simulink model "prochazkaModelWithVM"  (R2022b)
settings: Solver=VariableStepAuto  StartTime=0.0  StopTime=10.0  MaxStep=0.2  RelTol=1e-3
settings Model: SimulationMode=accelerator  Creator=migpa  LastModifiedBy=migpa
settings SolverCC: AlgebraicLoopSolver=TrustRegion
settings DebuggingCC: UnconnectedInputMsg=warning  UnconnectedOutputMsg=warning  UnconnectedLineMsg=warning  SFMachineParentedDataDiag=warning
settings ModelReferenceCC: EnableRefExpFcnMdlSchedulingChecks=on
settings RTWCC: DLArmComputeVersion=19.05

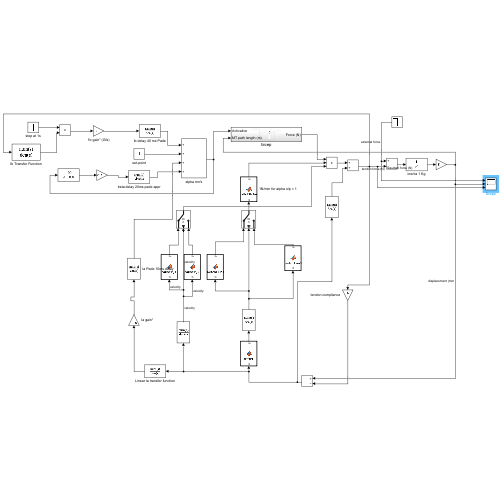
[thumbnail: Simulink's stored preview of the top-level diagram]
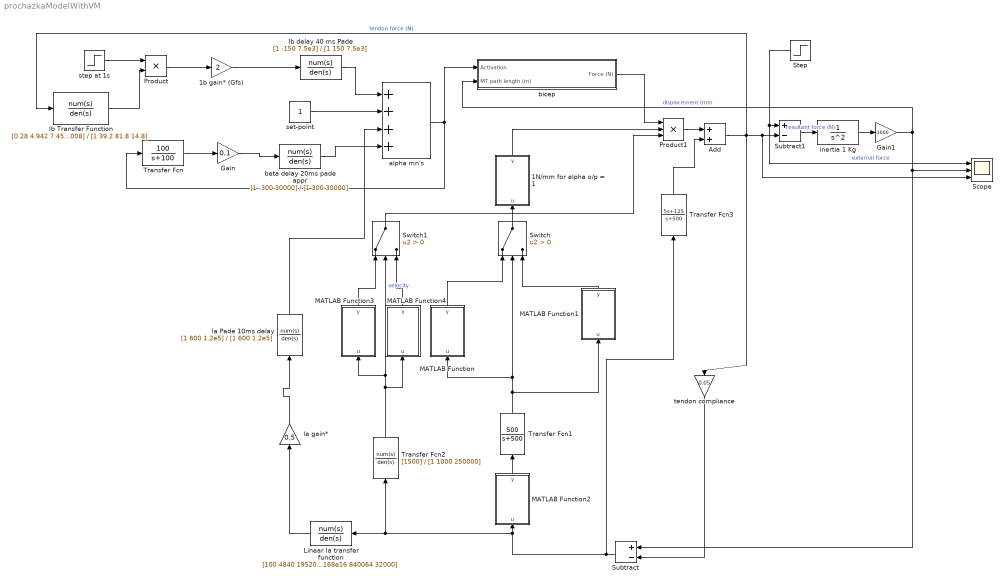
== system prochazkaModelWithVM ==
  1N/mm for alpha o/p = 1 : MATLAB Function  TreatAsAtomicUnit=on
  1b gain* (Gfs) : Gain  Gain=2
  Add : Sum
  Gain : Gain  Gain=0.1
  Gain1 : Gain  Gain=1000
  Ia Pade 10ms delay : TransferFcn  Numerator=[1 600 1.2e5]  Denominator=[1 600 1.2e5]
  Ia gain* : Gain  Gain=0.5
  Ib Transfer Function : TransferFcn  Numerator=[0.28 4.942 7.455 1.008]  Denominator=[1 39.2 81.8 14.8]
  Ib delay 40 ms Pade : TransferFcn  Numerator=[1 -150 7.5e3]  Denominator=[1 150 7.5e3]
  Linear Ia transfer function : TransferFcn  Numerator=[100 4840 19520 7040]  Denominator=[1 2000.84 1.00168e16 840064 32000]
  MATLAB Function : MATLAB Function  TreatAsAtomicUnit=on
  MATLAB Function1 : MATLAB Function  TreatAsAtomicUnit=on
  MATLAB Function2 : MATLAB Function  TreatAsAtomicUnit=on
  MATLAB Function3 : MATLAB Function  TreatAsAtomicUnit=on
  MATLAB Function4 : MATLAB Function  TreatAsAtomicUnit=on
  Product : Product
  Product1 : Product  Inputs=3
  Scope : Scope  NumInputPorts=3
  Step : Step  Before=30  After=0  SampleTime=0
  Subtract : Sum  Inputs=+-
  Subtract1 : Sum  Inputs=+-
  Switch : Switch  Criteria=u2 > Threshold  SaturateOnIntegerOverflow=off  InputSameDT=off
  Switch1 : Switch  Criteria=u2 > Threshold  SaturateOnIntegerOverflow=off  InputSameDT=off
  Transfer Fcn : TransferFcn  Numerator=[100]  Denominator=[1 100]
  Transfer Fcn1 : TransferFcn  Numerator=[500]  Denominator=[1 500]
  Transfer Fcn2 : TransferFcn  Numerator=[1500]  Denominator=[1 1000 250000]
  Transfer Fcn3 : TransferFcn  Numerator=[5 125]  Denominator=[1 500]
  alpha mn's : Sum  Inputs=++++
  beta delay 20ms pade appr : TransferFcn  Numerator=[1 -300 30000]  Denominator=[1 300 30000]
  bicep : Subsystem
  inertia 1 Kg : TransferFcn  Denominator=[1 0 0]
  set-point : Constant
  step at 1s : Step  SampleTime=0
  tendon compliance : Gain  Gain=0.05
  wires:
  Transfer Fcn/1 -> Gain/1
  step at 1s/1 -> Product/1
  Ib Transfer Function/1 -> Product/2
  set-point/1 -> alpha mn's/2
  Product/1 -> 1b gain* (Gfs)/1
  1b gain* (Gfs)/1 -> Ib delay 40 ms Pade/1
  Gain/1 -> beta delay 20ms pade appr/1
  alpha mn's/1 -> bicep/1(Activation), Transfer Fcn/1
  Switch/1 -> 1N/mm for alpha o/p = 1/1(u)
  bicep/1(Force (N)) -> Product1/1
  MATLAB Function/1(y) -> Switch/1
  MATLAB Function1/1(y) -> Switch/3
  Transfer Fcn1/1 -> MATLAB Function1/1(u), MATLAB Function/1(u), Switch/2
  MATLAB Function2/1(y) -> Transfer Fcn1/1
  Subtract/1 -> Transfer Fcn2/1, Linear Ia transfer function/1, MATLAB Function2/1(u), Transfer Fcn3/1
  tendon compliance/1 -> Subtract/2
  Ia gain*/1 -> Ia Pade 10ms delay/1
  Linear Ia transfer function/1 -> Ia gain*/1
  Ia Pade 10ms delay/1 -> alpha mn's/3
  1N/mm for alpha o/p = 1/1(y) -> Product1/2
  Transfer Fcn2/1 -> MATLAB Function4/1(u), MATLAB Function3/1(u), Switch1/2  "velocity"
  MATLAB Function3/1(y) -> Switch1/1
  MATLAB Function4/1(y) -> Switch1/3
  Switch1/1 -> Product1/3
  Product1/1 -> Add/1
  Transfer Fcn3/1 -> Add/2
  Add/1 -> tendon compliance/1, Ib Transfer Function/1, Scope/3, Subtract1/2  "tendon force (N)"
  Subtract1/1 -> inertia 1 Kg/1  "resultant force (N)"
  inertia 1 Kg/1 -> Gain1/1
  Gain1/1 -> Subtract/1, Scope/2, bicep/2(MT path length (m))  "displacement (mm"
  Step/1 -> Scope/1, Subtract1/1  "external force"
  Ib delay 40 ms Pade/1 -> alpha mn's/1
  beta delay 20ms pade appr/1 -> alpha mn's/4

== system prochazkaModelWithVM/bicep ==
  Activation : Inport
  MT path length (m) : Inport  Port=2
  Convert m to cm : Gain  Gain=100
  Recruitment : Subsystem
  fascicles (CE & PE) : Subsystem
  muscle mass : Subsystem
  series elastic element : Subsystem
  Force (N) : Outport
  wires:
  MT path length (m)/1 -> Convert m to cm/1
  series elastic element/1(Fse (N)) -> muscle mass/2(Fse (N)), Force (N)/1
  fascicles (CE & PE)/1(Force (N)) -> muscle mass/1(Fce (N))
  muscle mass/2(Lce (L0)) -> fascicles (CE & PE)/2(Length (L0)), series elastic element/2(Lce (L0))
  muscle mass/1(Vce (L0/s)) -> fascicles (CE & PE)/3(Velocity (L0/s))
  Recruitment/1(Frequencies (f0.5)) -> fascicles (CE & PE)/1(Frequencies (f0.5))
  Convert m to cm/1 -> series elastic element/1(Path (cm)), muscle mass/3(Path length [for init] (cm))
  Activation/1 -> Recruitment/1(Activation)

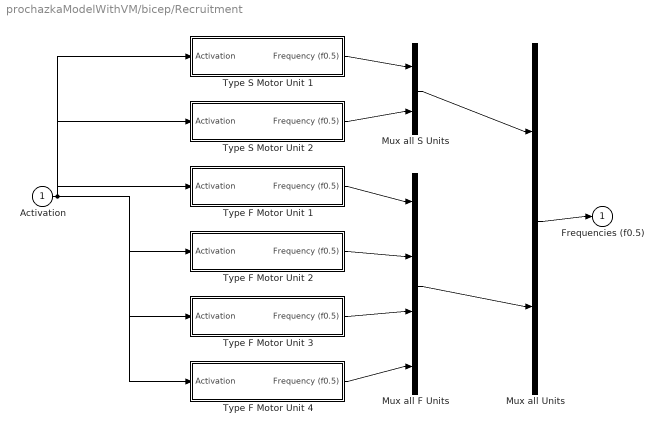
== system prochazkaModelWithVM/bicep/Recruitment ==
  Activation : Inport
  Mux all F Units : Mux
  Mux all S Units : Mux  Inputs=2
  Mux all Units : Mux  Inputs=2
  Type F Motor Unit 1 : Subsystem
  Type F Motor Unit 2 : Subsystem
  Type F Motor Unit 3 : Subsystem
  Type F Motor Unit 4 : Subsystem
  Type S Motor Unit 1 : Subsystem
  Type S Motor Unit 2 : Subsystem
  Frequencies (f0.5) : Outport
  wires:
  Activation/1 -> Type S Motor Unit 1/1(Activation), Type S Motor Unit 2/1(Activation), Type F Motor Unit 1/1(Activation), Type F Motor Unit 2/1(Activation), Type F Motor Unit 3/1(Activation), Type F Motor Unit 4/1(Activation)
  Type S Motor Unit 1/1(Frequency (f0.5)) -> Mux all S Units/1
  Type S Motor Unit 2/1(Frequency (f0.5)) -> Mux all S Units/2
  Mux all S Units/1 -> Mux all Units/1
  Type F Motor Unit 1/1(Frequency (f0.5)) -> Mux all F Units/1
  Type F Motor Unit 2/1(Frequency (f0.5)) -> Mux all F Units/2
  Type F Motor Unit 3/1(Frequency (f0.5)) -> Mux all F Units/3
  Type F Motor Unit 4/1(Frequency (f0.5)) -> Mux all F Units/4
  Mux all F Units/1 -> Mux all Units/2
  Mux all Units/1 -> Frequencies (f0.5)/1

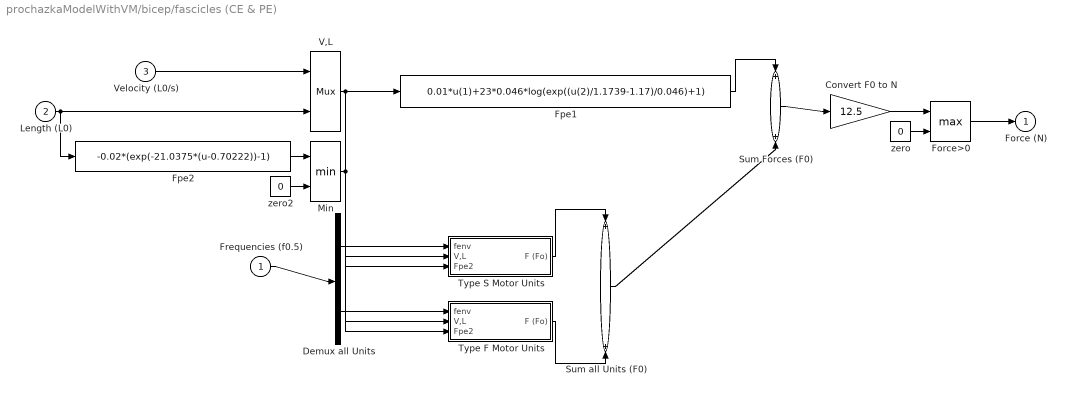
== system prochazkaModelWithVM/bicep/fascicles (CE & PE) ==
  Frequencies (f0.5) : Inport
  Length (L0) : Inport  Port=2
  Velocity (L0/s) : Inport  Port=3
  Convert F0 to N : Gain  Gain=12.5
  Demux all Units : Demux  Outputs="[2  4]"
  Force>0 : MinMax  Function=max  Inputs=2
  Fpe1 : Fcn  Expr=0.01*u(1)+23*0.046*log(exp((u(2)/1.1739-1.17)/0.046)+1)
  Fpe2 : Fcn  Expr=-0.02*(exp(-21.0375*(u-0.70222))-1)
  Min : MinMax  Inputs=2
  Sum Forces (F0) : Sum  Inputs=2
  Sum all Units (F0) : Sum
  Type F Motor Units : Subsystem
  Type S Motor Units : Subsystem
  V,L : Mux  Inputs=2
  zero : Constant  Value=0
  zero2 : Constant  Value=0
  Force (N) : Outport
  wires:
  Demux all Units/1 -> Type S Motor Units/1(fenv)
  V,L/1 -> Type S Motor Units/2(V,L), Type F Motor Units/2(V,L), Fpe1/1
  Min/1 -> Type S Motor Units/3(Fpe2), Type F Motor Units/3(Fpe2)
  Type S Motor Units/1(F (Fo)) -> Sum all Units (F0)/1
  Demux all Units/2 -> Type F Motor Units/1(fenv)
  Type F Motor Units/1(F (Fo)) -> Sum all Units (F0)/2
  Length (L0)/1 -> Fpe2/1, V,L/2
  Velocity (L0/s)/1 -> V,L/1
  Fpe2/1 -> Min/1
  zero2/1 -> Min/2
  Frequencies (f0.5)/1 -> Demux all Units/1
  Convert F0 to N/1 -> Force>0/1
  zero/1 -> Force>0/2
  Force>0/1 -> Force (N)/1
  Fpe1/1 -> Sum Forces (F0)/1
  Sum all Units (F0)/1 -> Sum Forces (F0)/2
  Sum Forces (F0)/1 -> Convert F0 to N/1

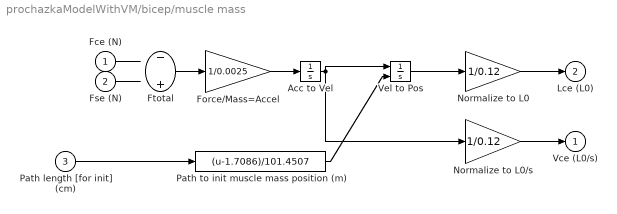
== system prochazkaModelWithVM/bicep/muscle mass ==
  Fce (N) : Inport
  Fse (N) : Inport  Port=2
  Path length [for init] (cm) : Inport  Port=3
  Acc to Vel : Integrator
  Force/Mass=Accel : Gain  Gain=1/0.0025
  Ftotal : Sum  Inputs=-+
  Normalize to L0 : Gain  Gain=1/0.12
  Normalize to L0/s : Gain  Gain=1/0.12
  Path to init muscle mass position (m) : Fcn  Expr=(u-1.7086)/101.4507
  Vel to Pos : Integrator  InitialConditionSource=external
  Vce (L0/s) : Outport
  Lce (L0) : Outport  Port=2
  wires:
  Ftotal/1 -> Force/Mass=Accel/1
  Force/Mass=Accel/1 -> Acc to Vel/1
  Acc to Vel/1 -> Vel to Pos/1, Normalize to L0/s/1
  Path length [for init] (cm)/1 -> Path to init muscle mass position (m)/1
  Path to init muscle mass position (m)/1 -> Vel to Pos/2
  Vel to Pos/1 -> Normalize to L0/1
  Fce (N)/1 -> ?
  Normalize to L0/1 -> Lce (L0)/1
  Fse (N)/1 -> ?
  Normalize to L0/s/1 -> Vce (L0/s)/1

== system prochazkaModelWithVM/bicep/series elastic element ==
  Path (cm) : Inport
  Lce (L0) : Inport  Port=2
  Convert Lce to Lse : Sum  Inputs=+-
  Convert to N : Gain  Gain=12.5
  Convert to cm : Gain  Gain=12
  Fse : Fcn  Expr=27.8*0.0047*log(exp((u(1)-0.964)/0.0047)+1)
  Normalize to L0T : Gain  Gain=1/2
  Fse (N) : Outport
  wires:
  Fse/1 -> Convert to N/1
  Normalize to L0T/1 -> Fse/1
  Convert Lce to Lse/1 -> Normalize to L0T/1
  Convert to N/1 -> Fse (N)/1
  Lce (L0)/1 -> Convert to cm/1
  Convert to cm/1 -> ?
  Path (cm)/1 -> ?

== system prochazkaModelWithVM/bicep/Recruitment/Type F Motor Unit 1 ==
  Activation : Inport
  Reached recruitment threshold? : Switch  Threshold=0.5
  determine frequency : Fcn  Expr=((2-0.5)/(1-(0.5)))*(u(1)-(0.5))+0.5
  zero : Constant  Value=0
  Frequency (f0.5) : Outport
  wires:
  Activation/1 -> Reached recruitment threshold?/2, determine frequency/1
  Reached recruitment threshold?/1 -> Frequency (f0.5)/1
  determine frequency/1 -> Reached recruitment threshold?/1
  zero/1 -> Reached recruitment threshold?/3

== system prochazkaModelWithVM/bicep/Recruitment/Type F Motor Unit 2 ==
  Activation : Inport
  Reached recruitment threshold? : Switch  Threshold=0.6
  determine frequency : Fcn  Expr=((2-0.5)/(1-(0.6)))*(u(1)-(0.6))+0.5
  zero : Constant  Value=0
  Frequency (f0.5) : Outport
  wires:
  Activation/1 -> Reached recruitment threshold?/2, determine frequency/1
  Reached recruitment threshold?/1 -> Frequency (f0.5)/1
  determine frequency/1 -> Reached recruitment threshold?/1
  zero/1 -> Reached recruitment threshold?/3

== system prochazkaModelWithVM/bicep/Recruitment/Type F Motor Unit 3 ==
  Activation : Inport
  Reached recruitment threshold? : Switch  Threshold=0.7
  determine frequency : Fcn  Expr=((2-0.5)/(1-(0.7)))*(u(1)-(0.7))+0.5
  zero : Constant  Value=0
  Frequency (f0.5) : Outport
  wires:
  Activation/1 -> Reached recruitment threshold?/2, determine frequency/1
  Reached recruitment threshold?/1 -> Frequency (f0.5)/1
  determine frequency/1 -> Reached recruitment threshold?/1
  zero/1 -> Reached recruitment threshold?/3

== system prochazkaModelWithVM/bicep/Recruitment/Type F Motor Unit 4 ==
  Activation : Inport
  Reached recruitment threshold? : Switch  Threshold=0.8
  determine frequency : Fcn  Expr=((2-0.5)/(1-(0.8)))*(u(1)-(0.8))+0.5
  zero : Constant  Value=0
  Frequency (f0.5) : Outport
  wires:
  Activation/1 -> Reached recruitment threshold?/2, determine frequency/1
  Reached recruitment threshold?/1 -> Frequency (f0.5)/1
  determine frequency/1 -> Reached recruitment threshold?/1
  zero/1 -> Reached recruitment threshold?/3

== system prochazkaModelWithVM/bicep/Recruitment/Type S Motor Unit 1 ==
  Activation : Inport
  Reached recruitment threshold? : Switch  Threshold=0.2
  determine frequency : Fcn  Expr=((2-0.5)/(1-(0.2)))*(u(1)-(0.2))+0.5
  zero : Constant  Value=0
  Frequency (f0.5) : Outport
  wires:
  Activation/1 -> Reached recruitment threshold?/2, determine frequency/1
  Reached recruitment threshold?/1 -> Frequency (f0.5)/1
  determine frequency/1 -> Reached recruitment threshold?/1
  zero/1 -> Reached recruitment threshold?/3

== system prochazkaModelWithVM/bicep/Recruitment/Type S Motor Unit 2 ==
  Activation : Inport
  Reached recruitment threshold? : Switch  Threshold=0.4
  determine frequency : Fcn  Expr=((2-0.5)/(1-(0.4)))*(u(1)-(0.4))+0.5
  zero : Constant  Value=0
  Frequency (f0.5) : Outport
  wires:
  Activation/1 -> Reached recruitment threshold?/2, determine frequency/1
  Reached recruitment threshold?/1 -> Frequency (f0.5)/1
  determine frequency/1 -> Reached recruitment threshold?/1
  zero/1 -> Reached recruitment threshold?/3

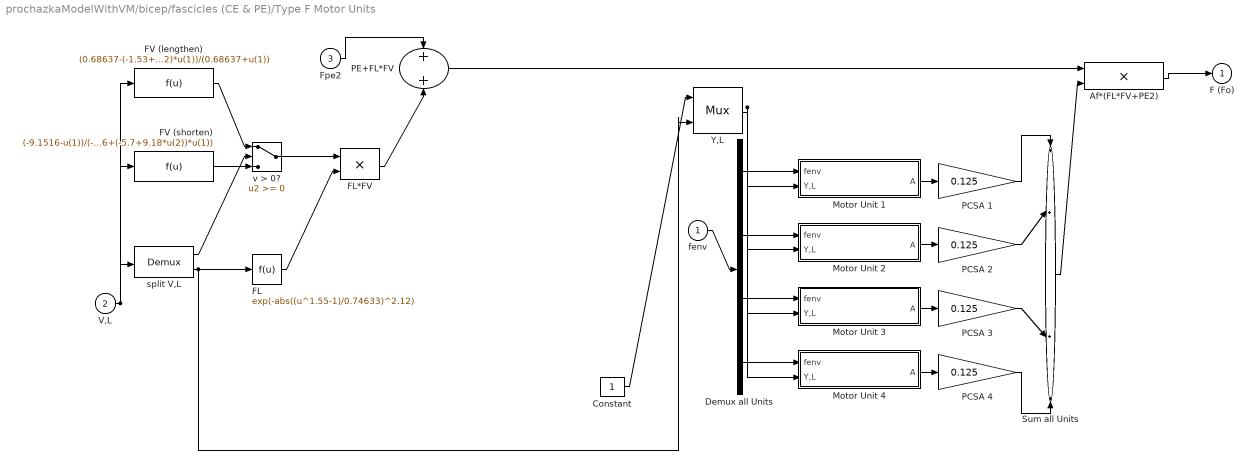
== system prochazkaModelWithVM/bicep/fascicles (CE & PE)/Type F Motor Units ==
  fenv : Inport
  V,L : Inport  Port=2
  Fpe2 : Inport  Port=3
  Af*(FL*FV+PE2) : Product
  Constant : Constant
  Demux all Units : Demux
  FL : Fcn  Expr=exp(-abs((u^1.55-1)/0.74633)^2.12)
  FL*FV : Product
  FV (lengthen) : Fcn  Expr=(0.68637-(-1.53+0*u(2)+0*u(2)^2)*u(1))/(0.68637+u(1))
  FV (shorten) : Fcn  Expr=(-9.1516-u(1))/(-9.1516+(-5.7+9.18*u(2))*u(1))
  Motor Unit 1 : Subsystem
  Motor Unit 2 : Subsystem
  Motor Unit 3 : Subsystem
  Motor Unit 4 : Subsystem
  PCSA {1..4} (4 alike) : Gain  Gain=0.125
  PE+FL*FV : Sum
  Sum all Units : Sum  Inputs=++++
  Y,L : Mux  Inputs=2
  split V,L : Demux  Outputs=2
  v > 0? : Switch
  F (Fo) : Outport
  wires:
  Constant/1 -> Y,L/1
  Y,L/1 -> Motor Unit 1/2(Y,L), Motor Unit 2/2(Y,L), Motor Unit 3/2(Y,L), Motor Unit 4/2(Y,L)
  Demux all Units/1 -> Motor Unit 1/1(fenv)
  Motor Unit 1/1(A) -> PCSA 1/1
  PCSA 1/1 -> Sum all Units/1
  Demux all Units/2 -> Motor Unit 2/1(fenv)
  Motor Unit 2/1(A) -> PCSA 2/1
  PCSA 2/1 -> Sum all Units/2
  Demux all Units/3 -> Motor Unit 3/1(fenv)
  Motor Unit 3/1(A) -> PCSA 3/1
  PCSA 3/1 -> Sum all Units/3
  Demux all Units/4 -> Motor Unit 4/1(fenv)
  Motor Unit 4/1(A) -> PCSA 4/1
  PCSA 4/1 -> Sum all Units/4
  Fpe2/1 -> PE+FL*FV/1
  V,L/1 -> FV (lengthen)/1, FV (shorten)/1, split V,L/1
  FV (lengthen)/1 -> v > 0?/1
  FV (shorten)/1 -> v > 0?/3
  split V,L/2 -> FL/1, Y,L/2
  FL/1 -> FL*FV/2
  split V,L/1 -> v > 0?/2
  v > 0?/1 -> FL*FV/1
  FL*FV/1 -> PE+FL*FV/2
  PE+FL*FV/1 -> Af*(FL*FV+PE2)/1
  fenv/1 -> Demux all Units/1
  Sum all Units/1 -> Af*(FL*FV+PE2)/2
  Af*(FL*FV+PE2)/1 -> F (Fo)/1

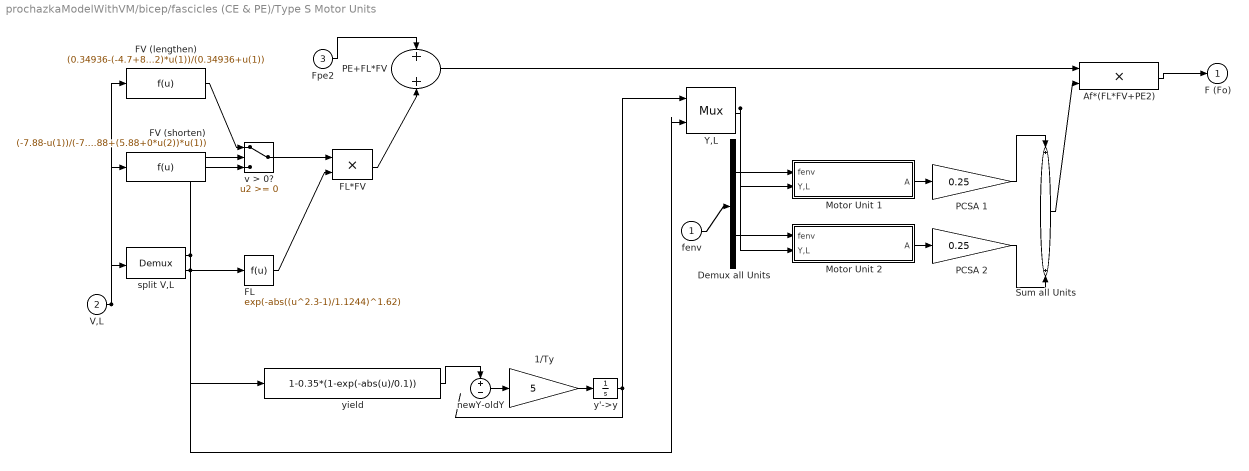
== system prochazkaModelWithVM/bicep/fascicles (CE & PE)/Type S Motor Units ==
  fenv : Inport
  V,L : Inport  Port=2
  Fpe2 : Inport  Port=3
  1/Ty : Gain  Gain=5
  Af*(FL*FV+PE2) : Product
  Demux all Units : Demux  Outputs=2
  FL : Fcn  Expr=exp(-abs((u^2.3-1)/1.1244)^1.62)
  FL*FV : Product
  FV (lengthen) : Fcn  Expr=(0.34936-(-4.7+8.41*u(2)+-5.31*u(2)^2)*u(1))/(0.34936+u(1))
  FV (shorten) : Fcn  Expr=(-7.88-u(1))/(-7.88+(5.88+0*u(2))*u(1))
  Motor Unit 1 : Subsystem
  Motor Unit 2 : Subsystem
  PCSA 1 : Gain  Gain=0.25
  PCSA 2 : Gain  Gain=0.25
  PE+FL*FV : Sum
  Sum all Units : Sum
  Y,L : Mux  Inputs=2
  newY-oldY : Sum  Inputs=+-
  split V,L : Demux  Outputs=2
  v > 0? : Switch
  y'->y : Integrator  InitialCondition=1
  yield : Fcn  Expr=1-0.35*(1-exp(-abs(u)/0.1))
  F (Fo) : Outport
  wires:
  split V,L/1 -> yield/1, v > 0?/2
  yield/1 -> newY-oldY/1
  newY-oldY/1 -> 1/Ty/1
  1/Ty/1 -> y'->y/1
  y'->y/1 -> Y,L/1
  Y,L/1 -> Motor Unit 1/2(Y,L), Motor Unit 2/2(Y,L)
  Demux all Units/1 -> Motor Unit 1/1(fenv)
  Motor Unit 1/1(A) -> PCSA 1/1
  PCSA 1/1 -> Sum all Units/1
  Demux all Units/2 -> Motor Unit 2/1(fenv)
  Motor Unit 2/1(A) -> PCSA 2/1
  PCSA 2/1 -> Sum all Units/2
  Fpe2/1 -> PE+FL*FV/1
  V,L/1 -> FV (lengthen)/1, FV (shorten)/1, split V,L/1
  FV (lengthen)/1 -> v > 0?/1
  FV (shorten)/1 -> v > 0?/3
  split V,L/2 -> FL/1, Y,L/2
  FL/1 -> FL*FV/2
  v > 0?/1 -> FL*FV/1
  FL*FV/1 -> PE+FL*FV/2
  PE+FL*FV/1 -> Af*(FL*FV+PE2)/1
  fenv/1 -> Demux all Units/1
  Sum all Units/1 -> Af*(FL*FV+PE2)/2
  Af*(FL*FV+PE2)/1 -> F (Fo)/1

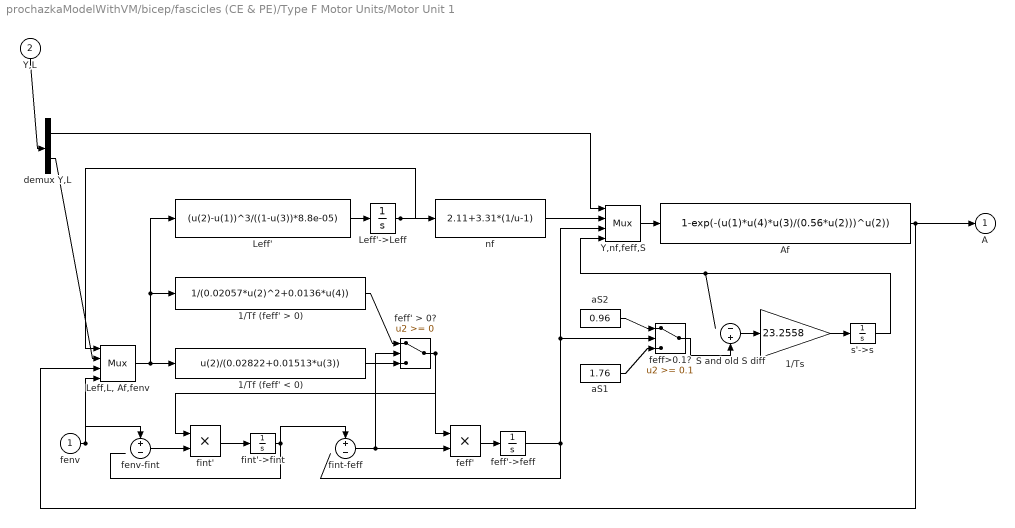
== system prochazkaModelWithVM/bicep/fascicles (CE & PE)/Type F Motor Units/Motor Unit 1 ==
  fenv : Inport
  Y,L : Inport  Port=2
  1/Tf (feff' < 0) : Fcn  Expr=u(2)/(0.02822+0.01513*u(3))
  1/Tf (feff' > 0) : Fcn  Expr=1/(0.02057*u(2)^2+0.0136*u(4))
  1/Ts : Gain  Gain=23.2558
  Af : Fcn  Expr=1-exp(-(u(1)*u(4)*u(3)/(0.56*u(2)))^u(2))
  Leff' : Fcn  Expr=(u(2)-u(1))^3/((1-u(3))*8.8e-05)
  Leff'->Leff : Integrator  InitialCondition=1
  "Leff,L, Af,fenv" : Mux
  S and old S diff : Sum  Inputs=-+
  Y,nf,feff,S : Mux
  aS1 : Constant  Value=1.76
  aS2 : Constant  Value=0.96
  demux Y,L : Demux  Outputs=2
  feff' : Product
  feff' > 0? : Switch
  feff'->feff : Integrator
  feff>0.1? : Switch  Threshold=0.1
  fenv-fint : Sum  Inputs=+-
  fint' : Product
  fint'->fint : Integrator
  fint-feff : Sum  Inputs=+-
  nf : Fcn  Expr=2.11+3.31*(1/u-1)
  s'->s : Integrator  InitialCondition=1.76
  A : Outport
  wires:
  Y,L/1 -> demux Y,L/1
  demux Y,L/1 -> Y,nf,feff,S/1
  demux Y,L/2 -> "Leff,L, Af,fenv"/2
  "Leff,L, Af,fenv"/1 -> 1/Tf (feff' < 0)/1, Leff'/1, 1/Tf (feff' > 0)/1
  1/Tf (feff' > 0)/1 -> feff' > 0?/1
  1/Tf (feff' < 0)/1 -> feff' > 0?/3
  fenv/1 -> fenv-fint/1, "Leff,L, Af,fenv"/4
  fenv-fint/1 -> fint'/2
  fint'/1 -> fint'->fint/1
  fint'->fint/1 -> fint-feff/1
  fint-feff/1 -> feff'/2, feff' > 0?/2
  feff' > 0?/1 -> feff'/1, fint'/1
  feff'/1 -> feff'->feff/1
  feff'->feff/1 -> Y,nf,feff,S/3, feff>0.1?/2
  Y,nf,feff,S/1 -> Af/1
  Af/1 -> "Leff,L, Af,fenv"/3, A/1
  Leff'/1 -> Leff'->Leff/1
  Leff'->Leff/1 -> "Leff,L, Af,fenv"/1, nf/1
  nf/1 -> Y,nf,feff,S/2
  aS2/1 -> feff>0.1?/1
  aS1/1 -> feff>0.1?/3
  feff>0.1?/1 -> S and old S diff/2
  S and old S diff/1 -> 1/Ts/1
  1/Ts/1 -> s'->s/1
  s'->s/1 -> Y,nf,feff,S/4

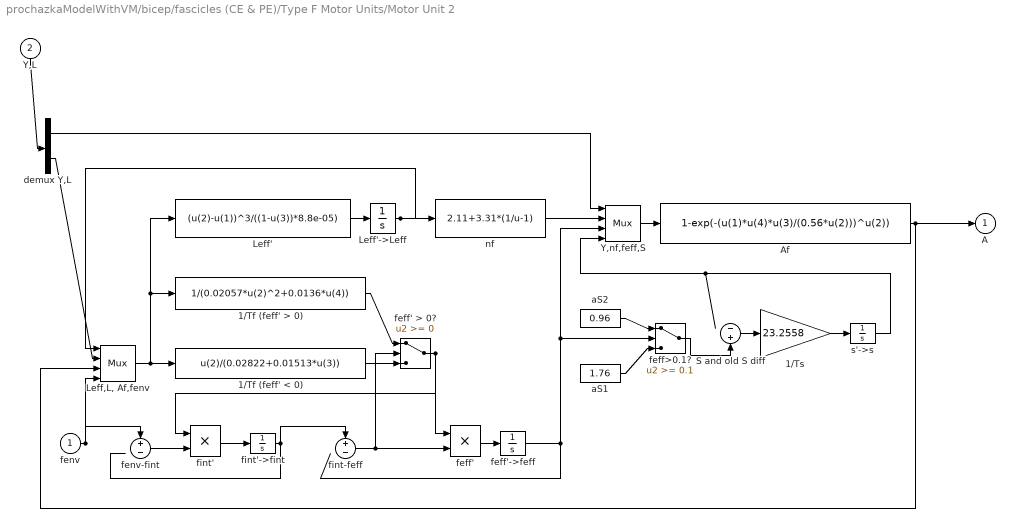
== system prochazkaModelWithVM/bicep/fascicles (CE & PE)/Type F Motor Units/Motor Unit 2 ==
  fenv : Inport
  Y,L : Inport  Port=2
  1/Tf (feff' < 0) : Fcn  Expr=u(2)/(0.02822+0.01513*u(3))
  1/Tf (feff' > 0) : Fcn  Expr=1/(0.02057*u(2)^2+0.0136*u(4))
  1/Ts : Gain  Gain=23.2558
  Af : Fcn  Expr=1-exp(-(u(1)*u(4)*u(3)/(0.56*u(2)))^u(2))
  Leff' : Fcn  Expr=(u(2)-u(1))^3/((1-u(3))*8.8e-05)
  Leff'->Leff : Integrator  InitialCondition=1
  "Leff,L, Af,fenv" : Mux
  S and old S diff : Sum  Inputs=-+
  Y,nf,feff,S : Mux
  aS1 : Constant  Value=1.76
  aS2 : Constant  Value=0.96
  demux Y,L : Demux  Outputs=2
  feff' : Product
  feff' > 0? : Switch
  feff'->feff : Integrator
  feff>0.1? : Switch  Threshold=0.1
  fenv-fint : Sum  Inputs=+-
  fint' : Product
  fint'->fint : Integrator
  fint-feff : Sum  Inputs=+-
  nf : Fcn  Expr=2.11+3.31*(1/u-1)
  s'->s : Integrator  InitialCondition=1.76
  A : Outport
  wires:
  Y,L/1 -> demux Y,L/1
  demux Y,L/1 -> Y,nf,feff,S/1
  demux Y,L/2 -> "Leff,L, Af,fenv"/2
  "Leff,L, Af,fenv"/1 -> 1/Tf (feff' < 0)/1, Leff'/1, 1/Tf (feff' > 0)/1
  1/Tf (feff' > 0)/1 -> feff' > 0?/1
  1/Tf (feff' < 0)/1 -> feff' > 0?/3
  fenv/1 -> fenv-fint/1, "Leff,L, Af,fenv"/4
  fenv-fint/1 -> fint'/2
  fint'/1 -> fint'->fint/1
  fint'->fint/1 -> fint-feff/1
  fint-feff/1 -> feff'/2, feff' > 0?/2
  feff' > 0?/1 -> feff'/1, fint'/1
  feff'/1 -> feff'->feff/1
  feff'->feff/1 -> Y,nf,feff,S/3, feff>0.1?/2
  Y,nf,feff,S/1 -> Af/1
  Af/1 -> "Leff,L, Af,fenv"/3, A/1
  Leff'/1 -> Leff'->Leff/1
  Leff'->Leff/1 -> "Leff,L, Af,fenv"/1, nf/1
  nf/1 -> Y,nf,feff,S/2
  aS2/1 -> feff>0.1?/1
  aS1/1 -> feff>0.1?/3
  feff>0.1?/1 -> S and old S diff/2
  S and old S diff/1 -> 1/Ts/1
  1/Ts/1 -> s'->s/1
  s'->s/1 -> Y,nf,feff,S/4

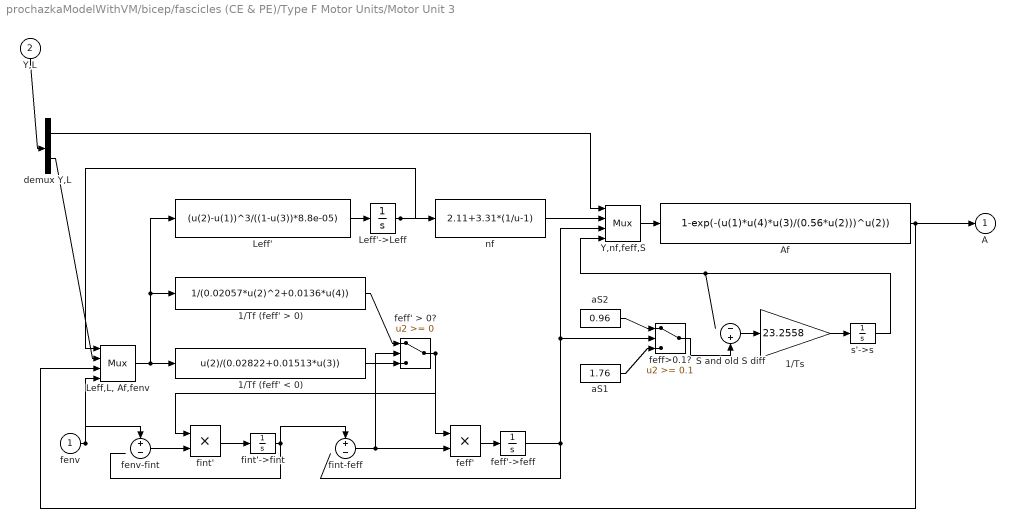
== system prochazkaModelWithVM/bicep/fascicles (CE & PE)/Type F Motor Units/Motor Unit 3 ==
  fenv : Inport
  Y,L : Inport  Port=2
  1/Tf (feff' < 0) : Fcn  Expr=u(2)/(0.02822+0.01513*u(3))
  1/Tf (feff' > 0) : Fcn  Expr=1/(0.02057*u(2)^2+0.0136*u(4))
  1/Ts : Gain  Gain=23.2558
  Af : Fcn  Expr=1-exp(-(u(1)*u(4)*u(3)/(0.56*u(2)))^u(2))
  Leff' : Fcn  Expr=(u(2)-u(1))^3/((1-u(3))*8.8e-05)
  Leff'->Leff : Integrator  InitialCondition=1
  "Leff,L, Af,fenv" : Mux
  S and old S diff : Sum  Inputs=-+
  Y,nf,feff,S : Mux
  aS1 : Constant  Value=1.76
  aS2 : Constant  Value=0.96
  demux Y,L : Demux  Outputs=2
  feff' : Product
  feff' > 0? : Switch
  feff'->feff : Integrator
  feff>0.1? : Switch  Threshold=0.1
  fenv-fint : Sum  Inputs=+-
  fint' : Product
  fint'->fint : Integrator
  fint-feff : Sum  Inputs=+-
  nf : Fcn  Expr=2.11+3.31*(1/u-1)
  s'->s : Integrator  InitialCondition=1.76
  A : Outport
  wires:
  Y,L/1 -> demux Y,L/1
  demux Y,L/1 -> Y,nf,feff,S/1
  demux Y,L/2 -> "Leff,L, Af,fenv"/2
  "Leff,L, Af,fenv"/1 -> 1/Tf (feff' < 0)/1, Leff'/1, 1/Tf (feff' > 0)/1
  1/Tf (feff' > 0)/1 -> feff' > 0?/1
  1/Tf (feff' < 0)/1 -> feff' > 0?/3
  fenv/1 -> fenv-fint/1, "Leff,L, Af,fenv"/4
  fenv-fint/1 -> fint'/2
  fint'/1 -> fint'->fint/1
  fint'->fint/1 -> fint-feff/1
  fint-feff/1 -> feff'/2, feff' > 0?/2
  feff' > 0?/1 -> feff'/1, fint'/1
  feff'/1 -> feff'->feff/1
  feff'->feff/1 -> Y,nf,feff,S/3, feff>0.1?/2
  Y,nf,feff,S/1 -> Af/1
  Af/1 -> "Leff,L, Af,fenv"/3, A/1
  Leff'/1 -> Leff'->Leff/1
  Leff'->Leff/1 -> "Leff,L, Af,fenv"/1, nf/1
  nf/1 -> Y,nf,feff,S/2
  aS2/1 -> feff>0.1?/1
  aS1/1 -> feff>0.1?/3
  feff>0.1?/1 -> S and old S diff/2
  S and old S diff/1 -> 1/Ts/1
  1/Ts/1 -> s'->s/1
  s'->s/1 -> Y,nf,feff,S/4

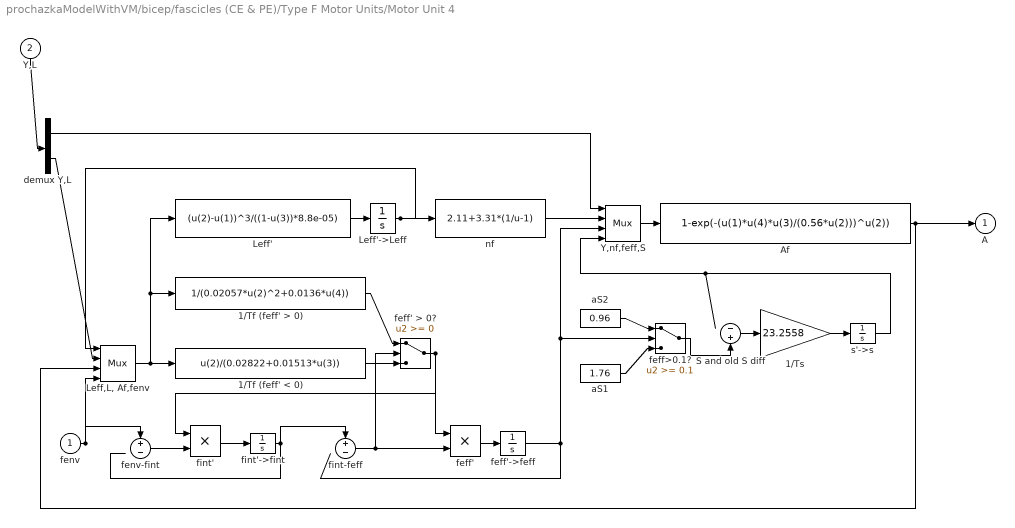
== system prochazkaModelWithVM/bicep/fascicles (CE & PE)/Type F Motor Units/Motor Unit 4 ==
  fenv : Inport
  Y,L : Inport  Port=2
  1/Tf (feff' < 0) : Fcn  Expr=u(2)/(0.02822+0.01513*u(3))
  1/Tf (feff' > 0) : Fcn  Expr=1/(0.02057*u(2)^2+0.0136*u(4))
  1/Ts : Gain  Gain=23.2558
  Af : Fcn  Expr=1-exp(-(u(1)*u(4)*u(3)/(0.56*u(2)))^u(2))
  Leff' : Fcn  Expr=(u(2)-u(1))^3/((1-u(3))*8.8e-05)
  Leff'->Leff : Integrator  InitialCondition=1
  "Leff,L, Af,fenv" : Mux
  S and old S diff : Sum  Inputs=-+
  Y,nf,feff,S : Mux
  aS1 : Constant  Value=1.76
  aS2 : Constant  Value=0.96
  demux Y,L : Demux  Outputs=2
  feff' : Product
  feff' > 0? : Switch
  feff'->feff : Integrator
  feff>0.1? : Switch  Threshold=0.1
  fenv-fint : Sum  Inputs=+-
  fint' : Product
  fint'->fint : Integrator
  fint-feff : Sum  Inputs=+-
  nf : Fcn  Expr=2.11+3.31*(1/u-1)
  s'->s : Integrator  InitialCondition=1.76
  A : Outport
  wires:
  Y,L/1 -> demux Y,L/1
  demux Y,L/1 -> Y,nf,feff,S/1
  demux Y,L/2 -> "Leff,L, Af,fenv"/2
  "Leff,L, Af,fenv"/1 -> 1/Tf (feff' < 0)/1, Leff'/1, 1/Tf (feff' > 0)/1
  1/Tf (feff' > 0)/1 -> feff' > 0?/1
  1/Tf (feff' < 0)/1 -> feff' > 0?/3
  fenv/1 -> fenv-fint/1, "Leff,L, Af,fenv"/4
  fenv-fint/1 -> fint'/2
  fint'/1 -> fint'->fint/1
  fint'->fint/1 -> fint-feff/1
  fint-feff/1 -> feff'/2, feff' > 0?/2
  feff' > 0?/1 -> feff'/1, fint'/1
  feff'/1 -> feff'->feff/1
  feff'->feff/1 -> Y,nf,feff,S/3, feff>0.1?/2
  Y,nf,feff,S/1 -> Af/1
  Af/1 -> "Leff,L, Af,fenv"/3, A/1
  Leff'/1 -> Leff'->Leff/1
  Leff'->Leff/1 -> "Leff,L, Af,fenv"/1, nf/1
  nf/1 -> Y,nf,feff,S/2
  aS2/1 -> feff>0.1?/1
  aS1/1 -> feff>0.1?/3
  feff>0.1?/1 -> S and old S diff/2
  S and old S diff/1 -> 1/Ts/1
  1/Ts/1 -> s'->s/1
  s'->s/1 -> Y,nf,feff,S/4

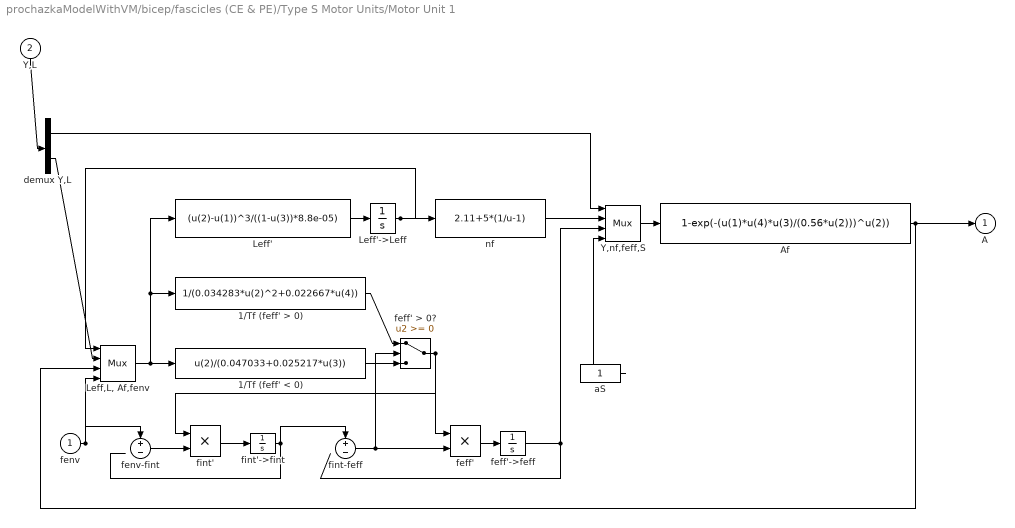
== system prochazkaModelWithVM/bicep/fascicles (CE & PE)/Type S Motor Units/Motor Unit 1 ==
  fenv : Inport
  Y,L : Inport  Port=2
  1/Tf (feff' < 0) : Fcn  Expr=u(2)/(0.047033+0.025217*u(3))
  1/Tf (feff' > 0) : Fcn  Expr=1/(0.034283*u(2)^2+0.022667*u(4))
  Af : Fcn  Expr=1-exp(-(u(1)*u(4)*u(3)/(0.56*u(2)))^u(2))
  Leff' : Fcn  Expr=(u(2)-u(1))^3/((1-u(3))*8.8e-05)
  Leff'->Leff : Integrator  InitialCondition=1
  "Leff,L, Af,fenv" : Mux
  Y,nf,feff,S : Mux
  aS : Constant
  demux Y,L : Demux  Outputs=2
  feff' : Product
  feff' > 0? : Switch
  feff'->feff : Integrator
  fenv-fint : Sum  Inputs=+-
  fint' : Product
  fint'->fint : Integrator
  fint-feff : Sum  Inputs=+-
  nf : Fcn  Expr=2.11+5*(1/u-1)
  A : Outport
  wires:
  Y,L/1 -> demux Y,L/1
  demux Y,L/1 -> Y,nf,feff,S/1
  demux Y,L/2 -> "Leff,L, Af,fenv"/2
  "Leff,L, Af,fenv"/1 -> 1/Tf (feff' < 0)/1, Leff'/1, 1/Tf (feff' > 0)/1
  1/Tf (feff' > 0)/1 -> feff' > 0?/1
  1/Tf (feff' < 0)/1 -> feff' > 0?/3
  fenv/1 -> fenv-fint/1, "Leff,L, Af,fenv"/4
  fenv-fint/1 -> fint'/2
  fint'/1 -> fint'->fint/1
  fint'->fint/1 -> fint-feff/1
  fint-feff/1 -> feff'/2, feff' > 0?/2
  feff' > 0?/1 -> feff'/1, fint'/1
  feff'/1 -> feff'->feff/1
  feff'->feff/1 -> Y,nf,feff,S/3
  Y,nf,feff,S/1 -> Af/1
  Af/1 -> "Leff,L, Af,fenv"/3, A/1
  Leff'/1 -> Leff'->Leff/1
  Leff'->Leff/1 -> "Leff,L, Af,fenv"/1, nf/1
  nf/1 -> Y,nf,feff,S/2
  aS/1 -> Y,nf,feff,S/4

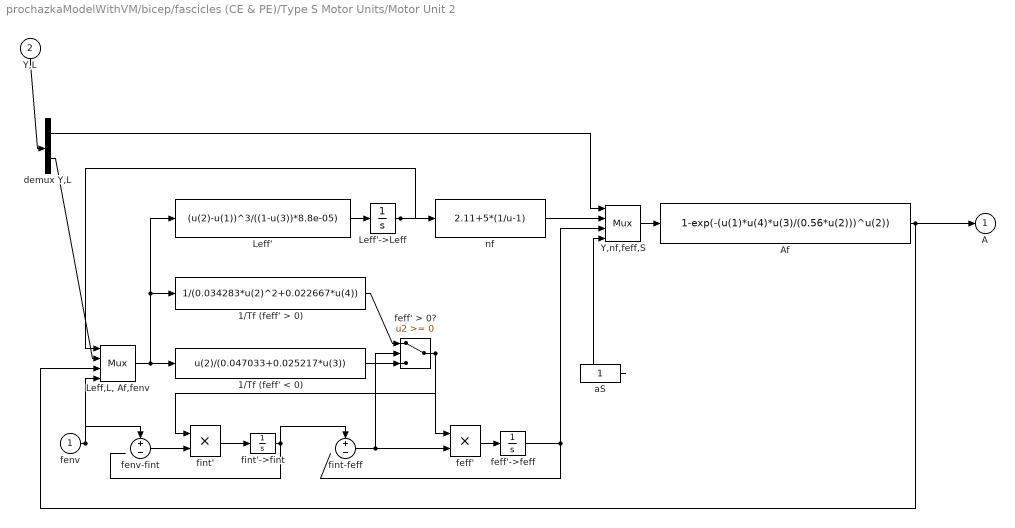
== system prochazkaModelWithVM/bicep/fascicles (CE & PE)/Type S Motor Units/Motor Unit 2 ==
  fenv : Inport
  Y,L : Inport  Port=2
  1/Tf (feff' < 0) : Fcn  Expr=u(2)/(0.047033+0.025217*u(3))
  1/Tf (feff' > 0) : Fcn  Expr=1/(0.034283*u(2)^2+0.022667*u(4))
  Af : Fcn  Expr=1-exp(-(u(1)*u(4)*u(3)/(0.56*u(2)))^u(2))
  Leff' : Fcn  Expr=(u(2)-u(1))^3/((1-u(3))*8.8e-05)
  Leff'->Leff : Integrator  InitialCondition=1
  "Leff,L, Af,fenv" : Mux
  Y,nf,feff,S : Mux
  aS : Constant
  demux Y,L : Demux  Outputs=2
  feff' : Product
  feff' > 0? : Switch
  feff'->feff : Integrator
  fenv-fint : Sum  Inputs=+-
  fint' : Product
  fint'->fint : Integrator
  fint-feff : Sum  Inputs=+-
  nf : Fcn  Expr=2.11+5*(1/u-1)
  A : Outport
  wires:
  Y,L/1 -> demux Y,L/1
  demux Y,L/1 -> Y,nf,feff,S/1
  demux Y,L/2 -> "Leff,L, Af,fenv"/2
  "Leff,L, Af,fenv"/1 -> 1/Tf (feff' < 0)/1, Leff'/1, 1/Tf (feff' > 0)/1
  1/Tf (feff' > 0)/1 -> feff' > 0?/1
  1/Tf (feff' < 0)/1 -> feff' > 0?/3
  fenv/1 -> fenv-fint/1, "Leff,L, Af,fenv"/4
  fenv-fint/1 -> fint'/2
  fint'/1 -> fint'->fint/1
  fint'->fint/1 -> fint-feff/1
  fint-feff/1 -> feff'/2, feff' > 0?/2
  feff' > 0?/1 -> feff'/1, fint'/1
  feff'/1 -> feff'->feff/1
  feff'->feff/1 -> Y,nf,feff,S/3
  Y,nf,feff,S/1 -> Af/1
  Af/1 -> "Leff,L, Af,fenv"/3, A/1
  Leff'/1 -> Leff'->Leff/1
  Leff'->Leff/1 -> "Leff,L, Af,fenv"/1, nf/1
  nf/1 -> Y,nf,feff,S/2
  aS/1 -> Y,nf,feff,S/4

== matlab function prochazkaModelWithVM/MATLAB Function ==
  data: u input; y output
function y = switchFun1(u)

y = 1-exp(-0.15*u);

== matlab function prochazkaModelWithVM/MATLAB Function2 ==
  data: u input; y output
function y = offset(u)

y = u-8;

== matlab function prochazkaModelWithVM/1N//mm for alpha o//p = 1 ==
  data: u input; y output
function y = parallelStiffness(u)

y = (10*u)+7;

== matlab function prochazkaModelWithVM/MATLAB Function3 ==
  data: u input; y output
function y = velocity1(u)

y = 1+(0.5*(1-exp(-1.5*u)));

== matlab function prochazkaModelWithVM/MATLAB Function4 ==
  data: u input; y output
function y = velocity2(u)

y = 1/(1-u);

== matlab function prochazkaModelWithVM/MATLAB Function1 ==
  data: u input; y output
function y = switchFun2(u)

y = -1+exp(0.15*u);
